simulink model "Dinamica_numerica_MPC"  (R2024b)
settings: Solver=ode4  StartTime=0.0  StopTime=Durata_sim  FixedStep=step_num  RelTol=1e-6
values from neighbouring files (symbols this model uses):
  a_c0 = 6771    [Propagation_outofplane_transfer.m]
  B_c = C_Dc*S_c/mass_c    (= 0)    [Propagation_outofplane_transfer.m]
  B_d = C_Dd*S_d/mass_d    (= 1.05e-08)    [Propagation_outofplane_transfer.m]
  D = zeros(ny,3)    [final_controller_1deputy2.m]
  delta_a0 = 0    [Propagation_outofplane_transfer.m]
  delta_B = (B_d-B_c)/B_d    (= 1)    [Propagation_outofplane_transfer.m]
  delta_e_x0 = 0    [Propagation_outofplane_transfer.m]
  delta_e_y0 = 0.2/a_c0    (= 2.95377344558e-05)    [Propagation_outofplane_transfer.m]
  delta_i_x0 = 0    [Propagation_outofplane_transfer.m]
  delta_i_y0 = 0.18/a_c0    (= 2.65839610102e-05)    [Propagation_outofplane_transfer.m]
  delta_lambda0 = 0    [Propagation_outofplane_transfer.m]
  e_c0 = 0.001    [Propagation_outofplane_transfer.m]
  i_c0 = 97.05 * pi/180    (= 1.69384203906)    [Propagation_outofplane_transfer.m]
  J_2 = 1.08263e-3    (= 0.00108263)    [Propagation_outofplane_transfer.m]
  M_c0 = 0 * pi/180    (= 0)    [Propagation_outofplane_transfer.m]
  mu = 3.986e5    (= 398600)    [Propagation_outofplane_transfer.m]
  OM_c0 = 30 * pi/180    (= 0.523598775598)    [Propagation_outofplane_transfer.m]
  om_c0 = 90 * pi/180    (= 1.57079632679)    [Propagation_outofplane_transfer.m]
  R_E = 6378    [Propagation_outofplane_transfer.m]
  rho = 1.05259630795205e-3    (= 0.00105259630795)    [Propagation_outofplane_transfer.m]
  ROE_T = [delta_aT,delta_lambdaT,delta_e_xT,delta_e_yT, delta_i_xT, delta_i_yT, delta_B]'    [Propagation_outofplane_transfer.m]
  S_c = 0.1*(1e-3)^2    (= 1e-07)    [Propagation_outofplane_transfer.m]
  S_d = 0.1*(1e-3)^2    (= 1e-07)    [Propagation_outofplane_transfer.m]
  T_orbit = 2*pi/n_c0    [Propagation_outofplane_transfer.m]
  Ts = 100    [Propagation_outofplane_transfer.m]
  u_max = max_thrust/mass_d    (= 3.25e-08)    [Propagation_outofplane_transfer.m]    (also in final_controller_1deputy2.m = 0.0325)
  u_min = min_thrust/mass_d    (= 1.75e-08)    [Propagation_outofplane_transfer.m]    (also in final_controller_1deputy2.m = 0.0175)
undefined symbols (not defined in the file or in its folder): final_controller_1deputy2, inputs4JB2008, JB2008, M_0, OMEGA_c0, omega_c0
libraries: spsMeanLib x6, simulink x3, simulink_extras x2
(part 4 of 4)

== matlab function Dinamica_numerica_MPC/matrix2columnvector ==
  data: M input; v output
function v = fcn(M)
v = rowwise_unroll(M);

== matlab function Dinamica_numerica_MPC/Calcolo rho e h/MATLAB Function ==
  data: t_UTC input; long output; geoc_lat output; norm_r_ECI output; r_ECI input; v_ECI input
function [long, geoc_lat, norm_r_ECI] = long_lat_h(t_UTC, r_ECI, v_ECI)
year_utc=t_UTC(1);
month_utc=t_UTC(2);
day_utc=t_UTC(3);
hour_utc=t_UTC(4);
min_utc=t_UTC(5);
sec_utc=t_UTC(6);
JD = MVS.date2JD(year_utc, month_utc, day_utc, hour_utc, min_utc, sec_utc);
JD2000=2451545;
alpha_G = JD2alphaG(JD, JD2000, year_utc,month_utc,day_utc,hour_utc,min_utc,sec_utc);
[r_ECEF, v_ECEF] = MVS.ECI2ECEF(r_ECI, v_ECI, alpha_G);
[geoc_lat, long] = ECEF2lat_lon(r_ECEF);
norm_r_ECI = norm(r_ECI,2);

== matlab function Dinamica_numerica_MPC/MATLAB Function1 ==
  data: R_E input; mu input; J_2 input; OE_c input; nu_c input; r_c_eci input; u_eci output; v_c_eci input; r_d_eci input; v_d_eci input; u_rtn input; r_rtn output
function [u_eci, r_rtn]  = compute_ECI_to_RTN(R_E,mu,J_2, OE_c, nu_c, r_c_eci,v_c_eci,r_d_eci,v_d_eci,u_rtn)

% Calcolo del vettore omega con il metodo del libro
a_c = OE_c(1);
e_c = OE_c(2);
i_c = OE_c(3);
OM_c = OE_c(4);
om_c = OE_c(5);
M_c = OE_c(6);
theta_c=om_c+nu_c;
h_vec = cross(r_c_eci, v_c_eci);
h = norm(h_vec,2);
r_c = norm(r_c_eci,2);
x_axis_rtn=r_c_eci/r_c;
z_axis_rtn=h_vec/h;
y_axis_rtn=cross(z_axis_rtn,x_axis_rtn);
om_z_rtn = h/r_c^2;
k_J2 = 3*J_2*mu*R_E^2/2;
om_x_rtn = -k_J2*sin(2*i_c)*sin(theta_c)/(h*r_c^3);
om_y_rtn = 0;
om_rtn = [om_x_rtn; om_y_rtn; om_z_rtn];
R =zeros(3,3);
R(1,1)=cos(theta_c)*cos(OM_c)-sin(theta_c)*cos(i_c)*sin(OM_c);
R(1,2) = -sin(theta_c)*cos(OM_c)-cos(theta_c)*cos(i_c)*sin(OM_c);
R(1,3)=sin(i_c)*sin(OM_c);
R(2,1)=cos(theta_c)*sin(OM_c)+sin(theta_c)*cos(i_c)*cos(OM_c);
R(2,2)=-sin(theta_c)*sin(OM_c)+cos(theta_c)*cos(i_c)*cos(OM_c);
R(2,3)=-sin(i_c)*cos(OM_c);
R(3,1)=sin(theta_c)*sin(i_c);
R(3,2)= cos(theta_c)*sin(i_c);
R(3,3)=cos(i_c);
om_eci1 = R*om_rtn;
om_eci2 = om_x_rtn*x_axis_rtn+om_z_rtn*z_axis_rtn;
differenza1 = om_eci1-om_eci2;
if any(abs(differenza1) > 1e-10)
    warning('I vettori velocità angolare calcolati con i 2 metodi sono diversi.');
end
L = [x_axis_rtn, y_axis_rtn, z_axis_rtn];
differenza2=R-L;
if any(abs(differenza2(:)) > 1e-6)
    warning('Le matrici DCM calcolate con i 2 metodi sono diverse.');
end


% Velocità angolare del frame LVLH rispetto a ECI (rad/s)

% om_eci=L*om_rtn;

% r_rtn=invL*(r_d_eci-r_c_eci);
% v_rtn=invL*v_d_eci-invL*v_c_eci-invL*cross(om_eci,L*r_rtn);
%----------------------------------------------------------

invR = R';
r_rtn=invR*(r_d_eci-r_c_eci);
v_rtn=invR*v_d_eci-invR*v_c_eci-invR*cross(om_eci2,R*r_rtn);

u_eci=R*u_rtn;
